simulink model "mainSimulink_localPi"  (R2021a)
settings: Solver=VariableStepAuto  StartTime=0.0  StopTime=20  FixedStep=samplingTime  RelTol=1e-3
model workspace (MATLAB code in the model file):
  | %% Simulink settings
  | controllerFile = 'directFFcontroller';
  | set_param('mainSimulink_localPi/Subsystem Reference', 'ReferencedSubsystem', controllerFile);
  | %% Display settings
  | scopeTimeSpan = 30;
  | 
  | %% Robot settings (must match Python)
  | sensorFreq = 125;
  | actuatorFreq = 250;
  | PiAddress = '131.155.230.140';
  | PiTCPport = 12345;
  | dataSize = 1;
  | sensorSamplingTime = 1/sensorFreq;
  | actuatorTime = 1/actuatorFreq;
  | actuatorMin = [0];                                  %Min relative pressure for actuators [kPa per actuator]
  | actuatorMax = [20];                                 %Max relative pressure for actuators [kPa per actuator]
  | regulatorMin = -100;                                %Min relative pressure output for regulators [kPa, same for all regulators]
  | regulatorMax = 100;                                 %Max relative pressure output for regulators [kPa, same for all regulators]
  | 
  | %% Unity communication settings (must match Unity)
  | UnityAddress = '127.0.0.1';                         %address for Matlab-Unity communication. 127.0.0.1 means local
  | UnityTCPport = 26950;                               %make sure that this port matches the one chosen in Unity
  | nrMessages = 1;                                     %nr of values that you are reading per packet. Depends on your Unity settings
  | UnitysampleFrequency = 120;                         %frequency on Simulink checking TCP connection
  | 
  | %%%ONLY EDIT WHEN THE UNITY MESSAGE TYPE OR HEADER CHANGES%%
  | headerWidth = 12;                                   %nr of bytes in message header (before actual message)
  | signalWidth = 8;                                    %length of each value in message, depends on data type (which is double for now, which is 8 bytes)
  | messageWidth = nrMessages .* signalWidth;           %length of message without header
  | totalMessageWidth = headerWidth + messageWidth;     %length of total packet
  | UnitySamplingTime = 1/UnitysampleFrequency;
values from neighbouring files (symbols this model uses):
  f = [1:0.02:7.02]    [Modulating_sine.m]
libraries: slrealtimeutilitieslib x4, slrealtimeiplib x2, instrumentlib x2
settings Model: Creator=chukh  LastModifiedBy=20210123

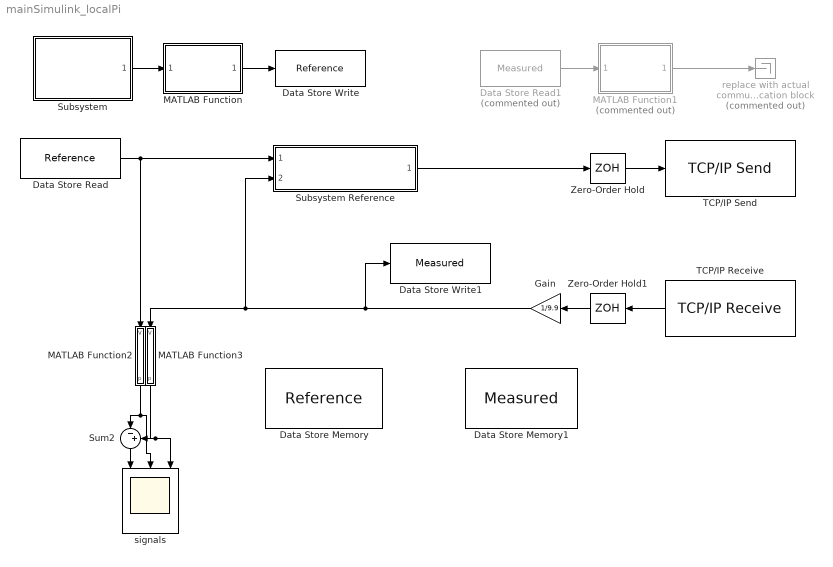
== system mainSimulink_localPi ==
  Data Store Memory : DataStoreMemory  DataStoreName=Reference  ReadBeforeWriteMsg=warning  WriteAfterWriteMsg=warning  WriteAfterReadMsg=warning  ShowAdditionalParam=off
  Data Store Memory1 : DataStoreMemory  DataStoreName=Measured  ReadBeforeWriteMsg=warning  WriteAfterWriteMsg=warning  WriteAfterReadMsg=warning  ShowAdditionalParam=off
  Data Store Read : DataStoreRead  DataStoreName=Reference  IndexOptions=Index vector (dialog)  Indices=1  OutputSizes=1
  Data Store Read1 : DataStoreRead  Commented=on  DataStoreName=Measured  IndexOptions=Index vector (dialog)  Indices=1  OutputSizes=1
  Data Store Write : DataStoreWrite  DataStoreName=Reference  IndexOptions=Index vector (dialog)  Indices=1  OutputSizes=1
  Data Store Write1 : DataStoreWrite  DataStoreName=Measured  IndexOptions=Index vector (dialog)  Indices=1  OutputSizes=1
  Gain : Gain  Gain=1/9.9
  MATLAB Function : MATLAB Function  TreatAsAtomicUnit=on
  MATLAB Function1 : MATLAB Function  Commented=on  TreatAsAtomicUnit=on
  MATLAB Function2 : MATLAB Function  TreatAsAtomicUnit=on
  MATLAB Function3 : MATLAB Function  TreatAsAtomicUnit=on
  Subsystem : Subsystem
  Subsystem Reference : Subsystem  ReferencedSubsystem=directFFcontroller
  Sum2 : Sum  Inputs=|-+
  TCP/IP Receive : instrumentlib/TCP//IP Receive  Host=PiAddress  Port=PiTCPport  DataSize=dataSize  EnableBlockingMode=on  Timeout=0.5  SampleTime=sensorSamplingTime  DataType=double  ByteOrder=LittleEndian  ASCIIFormatting=%f,  Terminator=LF
  TCP/IP Send : instrumentlib/TCP//IP Send  Host=PiAddress  Port=PiTCPport  EnableBlockingMode=on  Timeout=0.5  ByteOrder=LittleEndian  TransferDelay=on
  Zero-Order Hold : ZeroOrderHold  SampleTime=actuatorTime
  Zero-Order Hold1 : ZeroOrderHold  SampleTime=actuatorTime
  replace with actual communication block : Terminator  Commented=on
  signals : Scope  NumInputPorts=3
  wires:
  Subsystem Reference/1 -> Zero-Order Hold/1
  TCP/IP Receive/1 -> Zero-Order Hold1/1
  Zero-Order Hold/1 -> TCP/IP Send/1
  Zero-Order Hold1/1 -> Gain/1
  MATLAB Function2/1(p) -> Sum2/1, signals/2
  Gain/1 -> Data Store Write1/1, MATLAB Function3/1(V), Subsystem Reference/2
  MATLAB Function3/1(p) -> Sum2/2, signals/3
  Data Store Read/1 -> Subsystem Reference/1, MATLAB Function2/1(V)
  Sum2/1 -> signals/1
  Subsystem/1(" ") -> MATLAB Function/1(pressureFromUnity)
  MATLAB Function/1(pressureToPi) -> Data Store Write/1
  Data Store Read1/1 -> MATLAB Function1/1(pressureFromPi)
  MATLAB Function1/1(pressureToUnity) -> replace with actual communication block/1

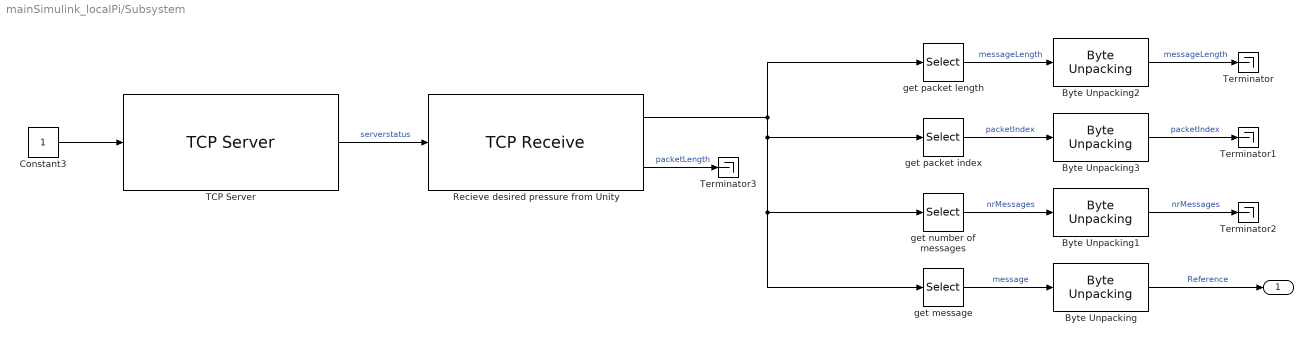
== system mainSimulink_localPi/Subsystem ==
  Byte Unpacking{,1..3} (4 alike) : slrealtimeutilitieslib/Byte Unpacking
      settings: SourceProductBaseCode=XP
  Constant3 : Constant  OutDataTypeStr=double
  Recieve desired pressure from Unity : slrealtimeiplib/TCP Receive  Priority=1  socketAddPortVal=Server: UnityAddress:UnityTCPport  rcvWidth=totalMessageWidth  sampleTime=UnitySamplingTime
      settings: SourceProductBaseCode=XP
  TCP Server : slrealtimeiplib/TCP Server  Priority=-1  useHostTargetConn=off  serverAddress=UnityAddress  serverPort=UnityTCPport
      settings: SourceProductBaseCode=XP
  Terminator{,1..3} (4 alike) : Terminator
  get message : Selector  InputPortWidth=totalMessageWidth  IndexOptions=Index vector (dialog)  Indices=[headerWidth+1:totalMessageWidth]  OutputSizes=1
  get number of messages : Selector  InputPortWidth=totalMessageWidth  IndexOptions=Index vector (dialog)  Indices=[signalWidth+1:headerWidth]  OutputSizes=1
  get packet index : Selector  InputPortWidth=totalMessageWidth  IndexOptions=Index vector (dialog)  Indices=[5:signalWidth]  OutputSizes=1
  get packet length : Selector  InputPortWidth=totalMessageWidth  IndexOptions=Index vector (dialog)  Indices=[1:4]  OutputSizes=1
  " " : Outport
  wires:
  TCP Server/1 -> Recieve desired pressure from Unity/1  "serverstatus"
  Recieve desired pressure from Unity/1 -> get packet index/1, get number of messages/1, get message/1, get packet length/1
  Byte Unpacking3/1 -> Terminator1/1  "packetIndex"
  get packet length/1 -> Byte Unpacking2/1  "messageLength"
  get number of messages/1 -> Byte Unpacking1/1  "nrMessages"
  Byte Unpacking1/1 -> Terminator2/1  "nrMessages"
  get packet index/1 -> Byte Unpacking3/1  "packetIndex"
  get message/1 -> Byte Unpacking/1  "message"
  Constant3/1 -> TCP Server/1
  Byte Unpacking2/1 -> Terminator/1  "messageLength"
  Byte Unpacking/1 -> " "/1  "Reference"
  Recieve desired pressure from Unity/2 -> Terminator3/1  "packetLength"

== matlab function mainSimulink_localPi/MATLAB Function2 ==
  data: V input; p output
function p = V2kPa(V)
p = (V-0.5)*200;

== matlab function mainSimulink_localPi/MATLAB Function3 ==
  data: V input; p output
function p = V2kPa(V)
p = (V-0.5)*200;

== matlab function mainSimulink_localPi/MATLAB Function1 ==
  data: pressureFromPi input; pressureToUnity output
function pressureToUnity = fcn(pressureFromPi)

pressureToUnity = zeros(1,nrMessages);                                %initialize with zeros

for c=1:nrMessages

minToPi = (actuatorMin(c) - regulatorMin) ./ (regulatorMax - regulatorMin);
maxToPi = (actuatorMax(c) - regulatorMin) ./ (regulatorMax - regulatorMin);
pressureToUnity(c) = (pressureFromPi(c) - minToPi) ./ (maxToPi - minToPi);

end

== matlab function mainSimulink_localPi/MATLAB Function ==
  data: pressureFromUnity input; pressureToPi output
function pressureToPi = fcn(pressureFromUnity)

zeroToPi = (0 - regulatorMin) ./ (regulatorMax - regulatorMin);
pressureToPi = repmat(zeroToPi,1,nrMessages); 

for c=1:nrMessages

    if(length(actuatorMin)~=dataSize)
       error('number of actuators does not match dataSize in Model Workspace'); 
    end
    
    if(pressureFromUnity(c) > 1)
       pressureFromUnity(c) = 1;
       warning('Unity is sending signals > 1');
    end
    
    if(pressureFromUnity(c) < 0)
       pressureFromUnity(c) = 0;
       warning('Unity is sending signals < 0');
    end

minToPi = (actuatorMin(c) - regulatorMin) ./ (regulatorMax - regulatorMin);
maxToPi = (actuatorMax(c) - regulatorMin) ./ (regulatorMax - regulatorMin);
    
pressureToPi(c) = minToPi + (maxToPi - minToPi).* pressureFromUnity(c);

end
